simulink model "model_constInput_noGen"  (R2021b)
settings: Solver=ode4  StartTime=0.0  StopTime=simOpt.SLmaxTime  FixedStep=simOpt.SLsmplTime  RelTol=1e-3
values from neighbouring files (symbols this model uses):
  D = D(ind_y,:)    [xpade.m]
undefined symbols (not defined in the file or in its folder): simOpt, SLin, strmatch
libraries: simulink x9, dspstat3 x3
settings Model: Creator=Hazim Namik  LastModifiedBy=puman
settings SolverCC: AlgebraicLoopSolver=LineSearch
settings DataIOCC: LimitDataPoints=on  SaveFormat=Array  SaveOutput=off  SignalLogging=off  SaveTime=off  SignalLoggingName=sigsOut
settings OptimizationCC: BlockReduction=off  BooleanDataType=off  LifeSpan=inf
settings DebuggingCC: SaveWithParameterizedLinksMsg=none  UnderspecifiedInitializationDetection=Classic  MergeDetectMultiDrivingBlocksExec=none  AllowSymbolicDim=off  PregeneratedLibrarySubsystemCodeDiagnostic=none  SFUnexpectedBacktrackingDiag=warning  SFNoUnconditionalDefaultTransitionDiag=warning  SFExecutionAtInitializationDiag=none  SFMachineParentedDataDiag=warning  ArithmeticOperatorsInVariantConditions=warning
settings HardwareCC: ProdBitPerPointer=32  ProdBitPerSizeT=32  ProdBitPerPtrDiffT=32  ProdLargestAtomicFloat=None  ProdIntDivRoundTo=Undefined  ProdEndianess=Unspecified  ProdWordSize=32  ProdHWDeviceType=32-bit Generic  TargetBitPerPointer=64  TargetBitPerSizeT=64  TargetBitPerPtrDiffT=64  TargetLongLongMode=on  TargetIntDivRoundTo=Zero  TargetEndianess=LittleEndian  TargetWordSize=64  TargetHWDeviceType=MATLAB Host  ProdEqTarget=off
settings ModelReferenceCC: PropagateSignalLabelsOutOfModel=off
settings SFSimCC: SimUseLocalCustomCode=off  CustomCodeUndefinedFunction=UseInterfaceOnly
settings RTWCC: RTWUseLocalCustomCode=off
settings CodeAppCC: StateflowObjectComments=on
settings GRTTargetCC: TargetLangStandard=C89/C90 (ANSI)
settings ConfigComp: CovMetricSettings=dw  CovSaveCumulativeToWorkspaceVar=on  CovSaveSingleToWorkspaceVar=on  CovExternalEMLEnable=off  CovSFcnEnable=off

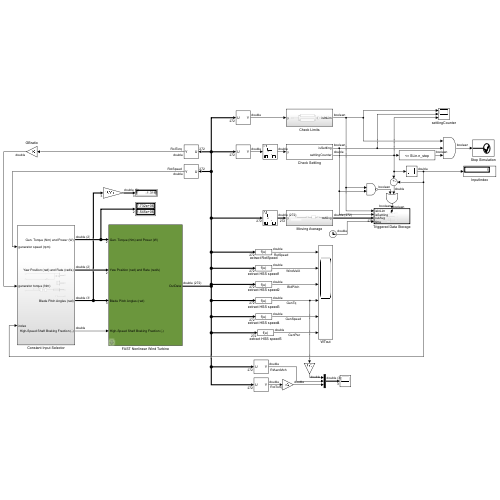
[thumbnail: Simulink's stored preview of the top-level diagram]
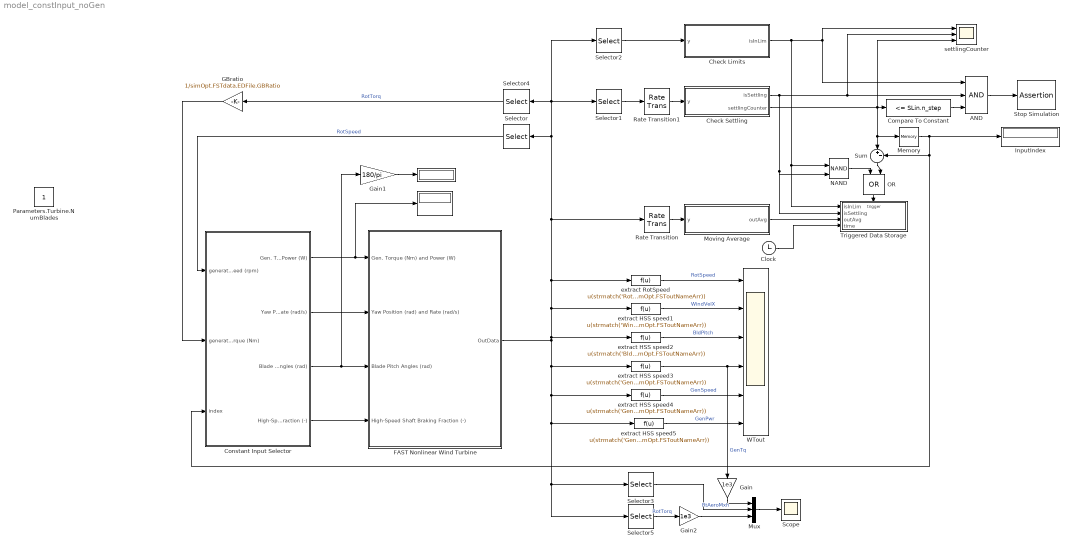
== system model_constInput_noGen ==
  " " : Display
  "  " : Display
  AND : Logic  Inputs=3  IconShape=distinctive  AllPortsSameDT=off  OutDataTypeStr=boolean
  Check Limits : Subsystem
  Check Settling : Subsystem
  Clock : Clock
  Compare To Constant : simulink/Logic and Bit Operations/Compare To Constant  relop=<=  const=SLin.n_step  OutDataTypeStr=boolean
  Constant Input Selector : Subsystem
  FAST Nonlinear Wind Turbine : Subsystem  mask(FAST Nonlinear Wind Turbine){}
      mask help: This block contains the FAST S-Function.
      mask init:
      | clear FAST_SFunc
  GBratio : Gain  Gain=1/simOpt.FSTdata.EDFile.GBRatio
  Gain : Gain  Gain=1e3
  Gain1 : Gain  Gain=180/pi
  Gain2 : Gain  Gain=1e3
  InputIndex : Display
  Memory : Memory  InitialCondition=1
  Moving Average : Subsystem
  Mux : Mux  Inputs=3
  NAND : Logic  Operator=NAND  IconShape=distinctive  AllPortsSameDT=off  OutDataTypeStr=boolean
  OR : Logic  Operator=OR  IconShape=distinctive  AllPortsSameDT=off  OutDataTypeStr=boolean
  Rate Transition : RateTransition
  Rate Transition1 : RateTransition
  Scope : Scope
  Selector : Selector  InputPortWidth=simOpt.n_out  IndexOptions=Index vector (dialog)  Indices=simOpt.idx.y.GenSpeed  OutputSizes=1
  Selector1 : Selector  InputPortWidth=simOpt.n_out  IndexOptions=Index vector (dialog)  Indices=simOpt.idx.y.settling  OutputSizes=1
  Selector2 : Selector  InputPortWidth=simOpt.n_out  IndexOptions=Index vector (dialog)  Indices=simOpt.idx.y.limCheck  OutputSizes=1
  Selector3 : Selector  InputPortWidth=simOpt.n_out  IndexOptions=Index vector (dialog)  Indices=simOpt.idx.y.RtAeroMxh  OutputSizes=1
  Selector4 : Selector  InputPortWidth=simOpt.n_out  IndexOptions=Index vector (dialog)  Indices=simOpt.idx.y.RotTorq  OutputSizes=1
  Selector5 : Selector  InputPortWidth=simOpt.n_out  IndexOptions=Index vector (dialog)  Indices=simOpt.idx.y.RotTorq  OutputSizes=1
  Stop Simulation : Assertion  AssertionFailFcn=set_param(bdroot,'SimulationCommand','stop')  StopWhenAssertionFail=off
  Sum : Sum  Inputs=|+-
  "Triggered Data Storage " : Subsystem  TreatAsAtomicUnit=on
  WTout : Scope  NumInputPorts=6
  extract HSS speed1 : Fcn  Expr=u(strmatch('Wind1VelX',simOpt.FSToutNameArr))
  extract HSS speed2 : Fcn  Expr=u(strmatch('BldPitch1',simOpt.FSToutNameArr))
  extract HSS speed3 : Fcn  Expr=u(strmatch('GenTq',simOpt.FSToutNameArr))
  extract HSS speed4 : Fcn  Expr=u(strmatch('GenSpeed',simOpt.FSToutNameArr))
  extract HSS speed5 : Fcn  Expr=u(strmatch('GenPwr',simOpt.FSToutNameArr))
  extract RotSpeed : Fcn  Expr=u(strmatch('RotSpeed',simOpt.FSToutNameArr))
  settlingCounter : Scope  NumInputPorts=3
  Parameters.Turbine.NumBlades : Constant  IOType=siggen
  wires:
  extract HSS speed1/1 -> WTout/2  "WindVelX"
  extract HSS speed2/1 -> WTout/3  "BldPitch"
  extract HSS speed3/1 -> WTout/4, Gain/1  "GenTq"
  extract HSS speed4/1 -> WTout/5  "GenSpeed"
  extract HSS speed5/1 -> WTout/6  "GenPwr"
  extract RotSpeed/1 -> WTout/1  "RotSpeed"
  Selector/1 -> Constant Input Selector/1(generator speed (rpm))  "RotSpeed"
  Selector1/1 -> Rate Transition1/1
  FAST Nonlinear Wind Turbine/1(OutData) -> Selector4/1, Selector2/1, Selector1/1, Selector/1, Rate Transition/1, extract RotSpeed/1, extract HSS speed1/1, extract HSS speed2/1, extract HSS speed4/1, Selector5/1, Selector3/1, extract HSS speed5/1, extract HSS speed3/1
  Rate Transition/1 -> Moving Average/1(y)
  Rate Transition1/1 -> Check Settling/1(y)
  Selector2/1 -> Check Limits/1(y)
  Check Limits/1(isInLim) -> NAND/1, "Triggered Data Storage "/1(isInLim), settlingCounter/1, AND/1
  Check Settling/1(isSettling) -> NAND/2, "Triggered Data Storage "/2(isSettling), settlingCounter/2, AND/2
  Moving Average/1(outAvg) -> "Triggered Data Storage "/3(outAvg)
  AND/1 -> Stop Simulation/1
  Compare To Constant/1 -> AND/3
  Clock/1 -> "Triggered Data Storage "/4(time)
  Check Settling/2(settlingCounter) -> Sum/1, Memory/1, settlingCounter/3, Compare To Constant/1
  Memory/1 -> InputIndex/1, Constant Input Selector/3(index), Sum/2
  Constant Input Selector/1(Gen. Torque (Nm) and Power (W)) -> "  "/1, FAST Nonlinear Wind Turbine/1(Gen. Torque (Nm) and Power (W))
  Constant Input Selector/2(Yaw Position (rad) and Rate (rad/s)) -> FAST Nonlinear Wind Turbine/2(Yaw Position (rad) and Rate (rad/s))
  Constant Input Selector/3(Blade Pitch Angles (rad)) -> Gain1/1, FAST Nonlinear Wind Turbine/3(Blade Pitch Angles (rad))
  Constant Input Selector/4(High-Speed Shaft Braking Fraction (-)) -> FAST Nonlinear Wind Turbine/4(High-Speed Shaft Braking Fraction (-))
  Gain1/1 -> " "/1
  OR/1 -> "Triggered Data Storage "/Trigger
  Sum/1 -> OR/2
  NAND/1 -> OR/1
  Mux/1 -> Scope/1
  Selector3/1 -> Mux/2  "RtAeroMxh"
  Gain/1 -> Mux/1
  Selector4/1 -> GBratio/1  "RotTorq"
  GBratio/1 -> Constant Input Selector/2(generator torque (Nm))
  Selector5/1 -> Gain2/1  "RotTorq"
  Gain2/1 -> Mux/3

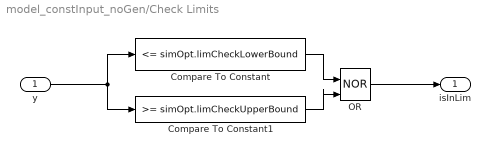
== system model_constInput_noGen/Check Limits ==
  y : Inport
  Compare To Constant : simulink/Logic and Bit Operations/Compare To Constant  relop=<=  const=simOpt.limCheckLowerBound  OutDataTypeStr=boolean
  Compare To Constant1 : simulink/Logic and Bit Operations/Compare To Constant  relop=>=  const=simOpt.limCheckUpperBound  OutDataTypeStr=boolean
  OR : Logic  Operator=NOR  IconShape=distinctive  AllPortsSameDT=off  OutDataTypeStr=boolean
  isInLim : Outport
  wires:
  y/1 -> Compare To Constant1/1, Compare To Constant/1
  OR/1 -> isInLim/1
  Compare To Constant1/1 -> OR/2
  Compare To Constant/1 -> OR/1

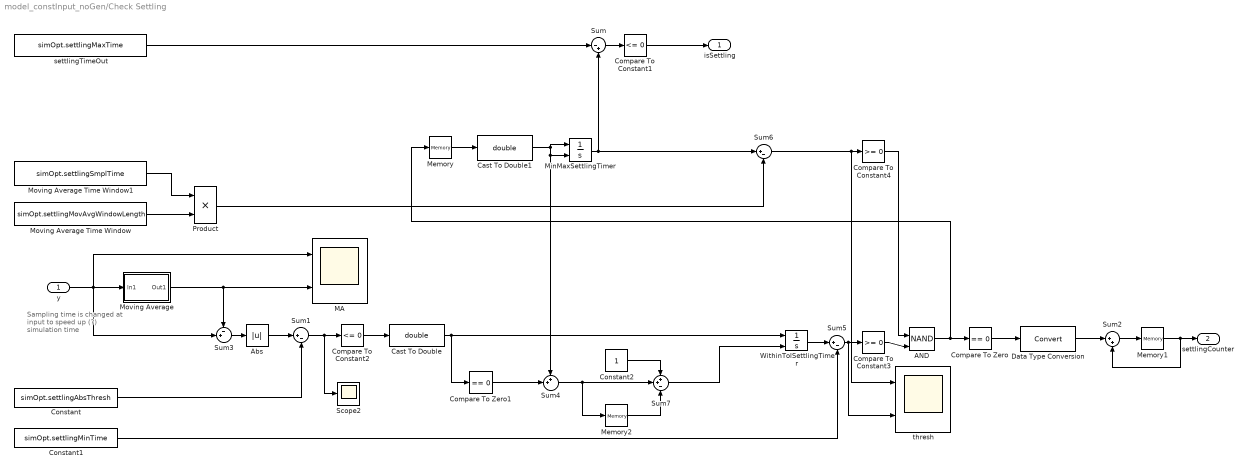
== system model_constInput_noGen/Check Settling ==
  note: Sampling time is changed at input
      | to speed up (?) simulation time
  y : Inport  SampleTime=simOpt.settlingSmplTime
  AND : Logic  Operator=NAND  IconShape=distinctive  AllPortsSameDT=off  OutDataTypeStr=boolean
  Abs : Abs
  Cast To Double : DataTypeConversion  OutDataTypeStr=double
  Cast To Double1 : DataTypeConversion  OutDataTypeStr=double
  Compare To Constant1 : simulink/Logic and Bit Operations/Compare To Constant  relop=<=  const=0  OutDataTypeStr=boolean
  Compare To Constant2 : simulink/Logic and Bit Operations/Compare To Constant  relop=<=  const=0  OutDataTypeStr=boolean
  Compare To Constant3 : simulink/Logic and Bit Operations/Compare To Constant  relop=>=  const=0  OutDataTypeStr=boolean
  Compare To Constant4 : simulink/Logic and Bit Operations/Compare To Constant  relop=>=  const=0  OutDataTypeStr=boolean
  Compare To Zero : simulink/Logic and Bit Operations/Compare To Zero  relop===  OutDataTypeStr=boolean
  Compare To Zero1 : simulink/Logic and Bit Operations/Compare To Zero  relop===  OutDataTypeStr=boolean
  Constant : Constant  Value=simOpt.settlingAbsThresh
  Constant1 : Constant  Value=simOpt.settlingMinTime
  Constant2 : Constant
  Data Type Conversion : DataTypeConversion
  MA : Scope  NumInputPorts=2
  Memory : Memory  InitialCondition=true
  Memory1 : Memory  InitialCondition=1  InheritSampleTime=on
  Memory2 : Memory  InitialCondition=1  InheritSampleTime=on
  MinMaxSettlingTimer : Integrator  ExternalReset=falling  LimitOutput=on  UpperSaturationLimit=max(simOpt.settlingMovAvgWindowLength*simOpt.settlingSmplTime,simOpt.settlingMaxTime)*1.01
  Moving Average : Subsystem
  Moving Average Time Window : Constant  Value=simOpt.settlingMovAvgWindowLength
  Moving Average Time Window1 : Constant  Value=simOpt.settlingSmplTime
  Product : Product
  Scope2 : Scope
  Sum : Sum  Inputs=|-+
  Sum1 : Sum  Inputs=|+-
  Sum2 : Sum  Inputs=|++
  Sum3 : Sum  Inputs=-+|
  Sum4 : Sum  Inputs=++|
  Sum5 : Sum  Inputs=|+-
  Sum6 : Sum  Inputs=|+-
  Sum7 : Sum  Inputs=++-
  WithinTolSettlingTimer : Integrator  ExternalReset=falling  LimitOutput=on  UpperSaturationLimit=simOpt.settlingMinTime
  settlingTimeOut : Constant  Value=simOpt.settlingMaxTime
  thresh : Scope  NumInputPorts=2
  isSettling : Outport
  settlingCounter : Outport  Port=2
  wires:
  AND/1 -> Compare To Zero/1, Memory/1
  MinMaxSettlingTimer/1 -> Sum6/1, Sum/2
  Sum6/1 -> thresh/1, Compare To Constant4/1
  Sum1/1 -> Scope2/1, Compare To Constant2/1
  WithinTolSettlingTimer/1 -> Sum5/1
  y/1 -> MA/1, Moving Average/1(In1), Sum3/2
  Abs/1 -> Sum1/1
  Sum3/1 -> Abs/1
  Sum5/1 -> thresh/2, Compare To Constant3/1
  Moving Average Time Window/1 -> Product/2
  Compare To Constant2/1 -> Cast To Double/1
  Constant/1 -> Sum1/2
  Constant1/1 -> Sum5/2
  Compare To Constant3/1 -> AND/2
  Compare To Constant4/1 -> AND/1
  Memory/1 -> Cast To Double1/1
  Cast To Double1/1 -> Sum4/1, MinMaxSettlingTimer/2, MinMaxSettlingTimer/1
  Moving Average/1(Out1) -> Sum3/1, MA/2
  settlingTimeOut/1 -> Sum/1
  Sum/1 -> Compare To Constant1/1
  Compare To Constant1/1 -> isSettling/1
  Memory1/1 -> settlingCounter/1, Sum2/2
  Sum2/1 -> Memory1/1
  Compare To Zero/1 -> Data Type Conversion/1
  Data Type Conversion/1 -> Sum2/1
  Moving Average Time Window1/1 -> Product/1
  Product/1 -> Sum6/2
  Sum7/1 -> WithinTolSettlingTimer/2
  Compare To Zero1/1 -> Sum4/2
  Cast To Double/1 -> WithinTolSettlingTimer/1, Compare To Zero1/1
  Sum4/1 -> Sum7/2, Memory2/1
  Memory2/1 -> Sum7/3
  Constant2/1 -> Sum7/1

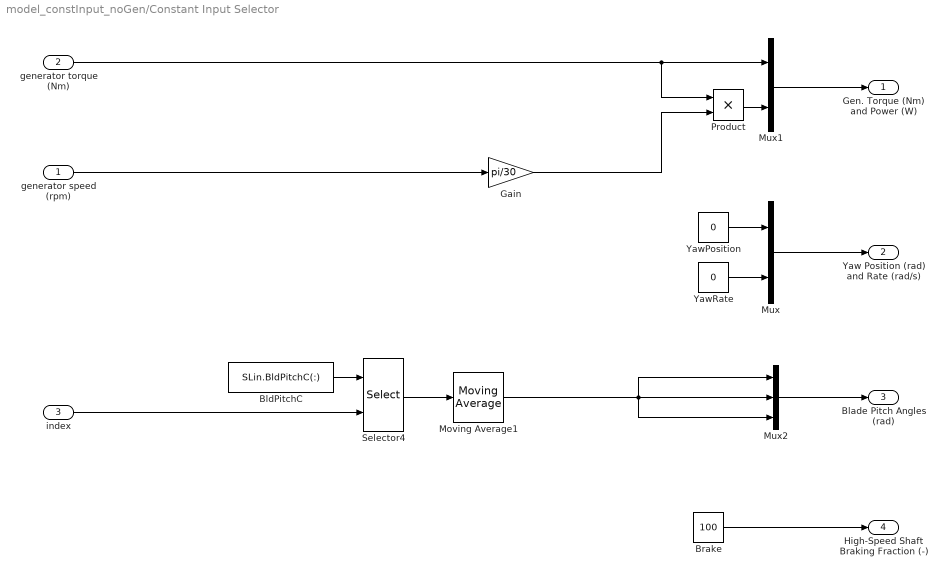
== system model_constInput_noGen/Constant Input Selector ==
  generator speed (rpm) : Inport
  generator torque (Nm) : Inport  Port=2
  index : Inport  Port=3
  BldPitchC : Constant  Value=SLin.BldPitchC(:)
  Brake : Constant  Value=100
  Gain : Gain  Gain=pi/30
  Moving Average1 : dspstat3/Moving Average  Method=Sliding window  ForgettingFactorPort=off  SpecifyWindowLength=on  WindowLength=8  ForgettingFactor=0.99  SimulateUsing=Interpreted execution
  Mux : Mux  Inputs=2
  Mux1 : Mux  Inputs=2
  Mux2 : Mux  Inputs=3
  Product : Product
  Selector4 : Selector  InputPortWidth=SLin.n_step  IndexOptions=Index vector (port)  Indices=simOpt.i_outRotSpeed  OutputSizes=1
  YawPosition : Constant  Value=0
  YawRate : Constant  Value=0
  Gen. Torque (Nm) and Power (W) : Outport
  Yaw Position (rad) and Rate (rad/s) : Outport  Port=2
  Blade Pitch Angles (rad) : Outport  Port=3
  High-Speed Shaft Braking Fraction (-) : Outport  Port=4
  wires:
  YawRate/1 -> Mux/2
  index/1 -> Selector4/2
  YawPosition/1 -> Mux/1
  BldPitchC/1 -> Selector4/1
  Product/1 -> Mux1/2
  Mux2/1 -> Blade Pitch Angles (rad)/1
  Brake/1 -> High-Speed Shaft Braking Fraction (-)/1
  generator speed (rpm)/1 -> Gain/1
  Mux1/1 -> Gen. Torque (Nm) and Power (W)/1
  Mux/1 -> Yaw Position (rad) and Rate (rad/s)/1
  Gain/1 -> Product/2
  generator torque (Nm)/1 -> Product/1, Mux1/1
  Selector4/1 -> Moving Average1/1
  Moving Average1/1 -> Mux2/1, Mux2/3, Mux2/2

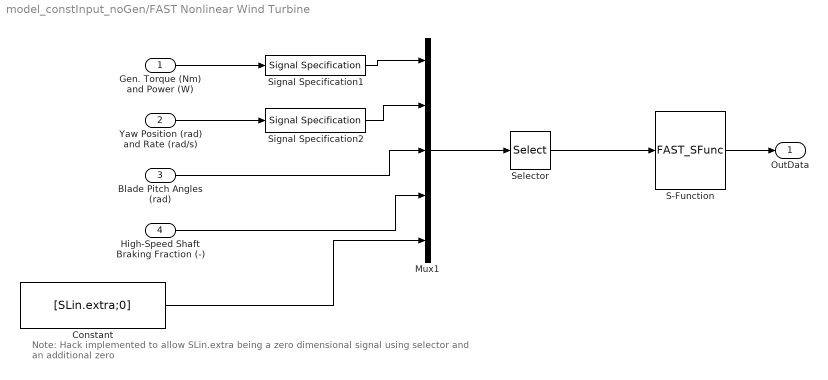
== system model_constInput_noGen/FAST Nonlinear Wind Turbine ==
  note: Note: Hack implemented to allow SLin.extra being a zero dimensional signal using selector and an additional zero
  Gen. Torque (Nm) and Power (W) : Inport
  Yaw Position (rad) and Rate (rad/s) : Inport  Port=2
  Blade Pitch Angles (rad) : Inport  Port=3
  High-Speed Shaft Braking Fraction (-) : Inport  Port=4
  Constant : Constant  Value=[SLin.extra;0]
  Mux1 : Mux  Inputs=5
  S-Function : S-Function  FunctionName=FAST_SFunc  Parameters=simOpt.FSTnewInputFile, simOpt.SLmaxTime, 0  SFunctionDeploymentMode=off  EnableBusSupport=off
  Selector : Selector  InputPortWidth=9+numel(SLin.extra)  IndexOptions=Index vector (dialog)  Indices=1:(8+numel(SLin.extra))  OutputSizes=1
  Signal Specification1 : SignalSpecification  OutDataTypeStr=double  Dimensions=2
  Signal Specification2 : SignalSpecification  OutDataTypeStr=double  Dimensions=2
  OutData : Outport  VectorParamsAs1DForOutWhenUnconnected=off
  wires:
  Gen. Torque (Nm) and Power (W)/1 -> Signal Specification1/1
  S-Function/1 -> OutData/1
  Mux1/1 -> Selector/1
  Blade Pitch Angles (rad)/1 -> Mux1/3
  Yaw Position (rad) and Rate (rad/s)/1 -> Signal Specification2/1
  Signal Specification1/1 -> Mux1/1
  Signal Specification2/1 -> Mux1/2
  High-Speed Shaft Braking Fraction (-)/1 -> Mux1/4
  Constant/1 -> Mux1/5
  Selector/1 -> S-Function/1

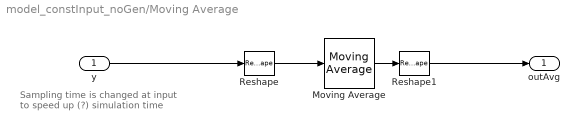
== system model_constInput_noGen/Moving Average ==
  note: Sampling time is changed at input
      | to speed up (?) simulation time
  y : Inport  SampleTime=simOpt.settlingSmplTime
  Moving Average : dspstat3/Moving Average  Method=Sliding window  ForgettingFactorPort=off  SpecifyWindowLength=on  WindowLength=simOpt.settlingMovAvgWindowLength  ForgettingFactor=0.99  SimulateUsing=Interpreted execution
  Reshape : Reshape  OutputDimensionality=Row vector (2-D)
  Reshape1 : Reshape
  outAvg : Outport
  wires:
  y/1 -> Reshape/1
  Moving Average/1 -> Reshape1/1
  Reshape/1 -> Moving Average/1
  Reshape1/1 -> outAvg/1

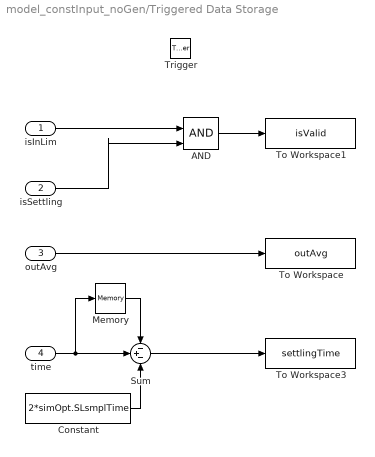
== system model_constInput_noGen/Triggered Data Storage  ==
  isInLim : Inport
  isSettling : Inport  Port=2
  outAvg : Inport  Port=3
  time : Inport  Port=4
  Trigger : TriggerPort  VariantControl=(inherit)
  AND : Logic  IconShape=distinctive  AllPortsSameDT=off  OutDataTypeStr=boolean
  Constant : Constant  Value=2*simOpt.SLsmplTime
  Memory : Memory  InheritSampleTime=on
  Sum : Sum  Inputs=-+-
  To Workspace : ToWorkspace  VariableName=outAvg  SampleTime=-1
  To Workspace1 : ToWorkspace  VariableName=isValid  SampleTime=-1
  To Workspace3 : ToWorkspace  VariableName=settlingTime  SampleTime=-1
  wires:
  outAvg/1 -> To Workspace/1
  isInLim/1 -> AND/1
  isSettling/1 -> AND/2
  Sum/1 -> To Workspace3/1
  time/1 -> Sum/2, Memory/1
  AND/1 -> To Workspace1/1
  Constant/1 -> Sum/3
  Memory/1 -> Sum/1

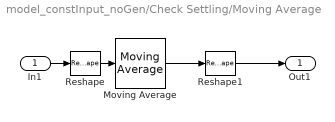
== system model_constInput_noGen/Check Settling/Moving Average ==
  In1 : Inport
  Moving Average : dspstat3/Moving Average  Method=Sliding window  ForgettingFactorPort=off  SpecifyWindowLength=on  WindowLength=simOpt.settlingMovAvgWindowLength  ForgettingFactor=0.99  SimulateUsing=Interpreted execution
  Reshape : Reshape  OutputDimensionality=Row vector (2-D)
  Reshape1 : Reshape
  Out1 : Outport
  wires:
  Moving Average/1 -> Reshape1/1
  Reshape1/1 -> Out1/1
  Reshape/1 -> Moving Average/1
  In1/1 -> Reshape/1
